simulink model "IMPexample2sim"  (R2018a)
settings: Solver=VariableStepAuto  StartTime=0.0  StopTime=10.0  RelTol=1e-3
values from neighbouring files (symbols this model uses):
  Ao = [Ap-Bp*Kp-Jp*Cp zeros(size(Ap,1),size(Av,2));-Jv*Cp Av]    [IMPexample2.m]
  Bo = [Jp Bp;Jv zeros(size(Jv,1),size(Bp,2))]    [IMPexample2.m]
  Bpo = [Jp Bp]    [IMPexample2.m]
  Jp = acker(Ap',Cp',-100)'    [IMPexample2.m]    (also in IMPexample3.m)
  Jv = acker(Av',Cv',[-10 -10 -10 -10])'    [IMPexample2.m]    (also in IMPexample3.m = acker(Av',Cv',[-10 -10 -10])')
  K = [Kp Cv]    [IMPexample2.m]
  Kp = acker(Ap,Bp,-10)    [IMPexample2.m]    (also in IMPexample3.m)
  Kpre = 1/evalfr(T,0)    [IMPexample2.m]    (also in IMPexample3.m)
  ref = 70*2*pi/60    (= 7.33038285838)    [IMPexample.m]    (also in IMPexample2.m; IMPexample3.m)
  Ts = 0.01    [IMPexample.m]    (also in IMPexample2.m)
undefined symbols (not defined in the file or in its folder): Ao_, Ap, Ap_, Apo_, Av, Avo_, Bo_, Bp, Bp_, Bpo_, Bvo_, Co_, Cp, Cp_, Cpo_, Cv, Cvo_, DiscIntNeverNeededParam, Do_, Dpo_, Dvo_, Jp_, Kp_
libraries: simulink x2
settings Model: Creator=Tobias Scala  LastModifiedBy=Tobias Scala

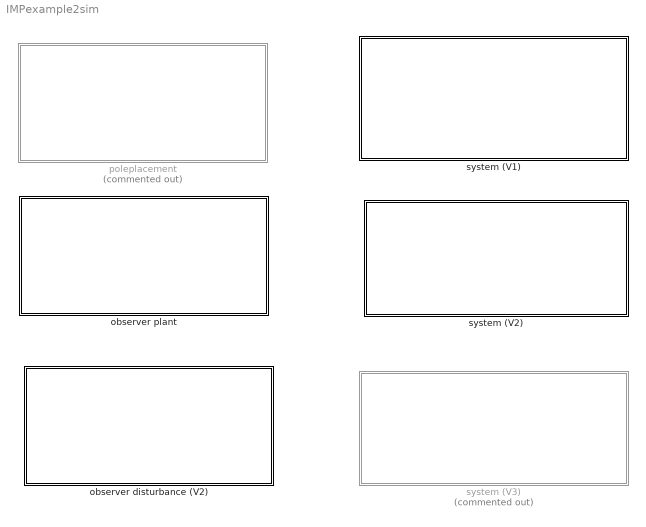
== system IMPexample2sim ==
  observer disturbance (V2) : Subsystem
  observer plant : Subsystem
  poleplacement : Subsystem  Commented=on
  system (V1) : Subsystem
  system (V2) : Subsystem
  system (V3) : Subsystem  Commented=on

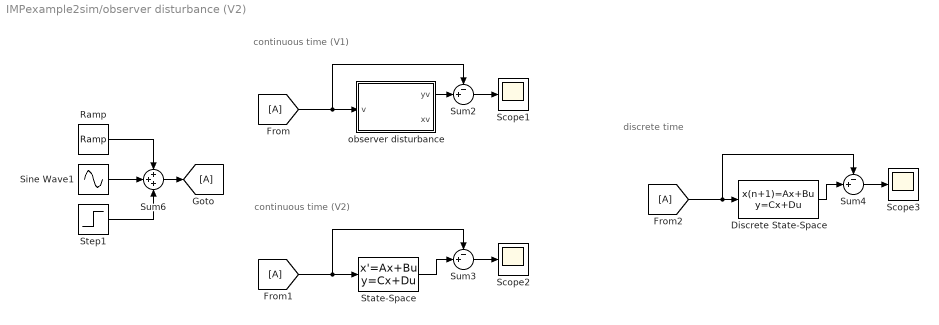
== system IMPexample2sim/observer disturbance (V2) ==
  note: discrete time
  note: continuous time (V2)
  note: continuous time (V1)
  Discrete State-Space : DiscreteStateSpace  A=Avo_  B=Bvo_  C=Cvo_  D=Dvo_  SampleTime=Ts
  Ramp : simulink/Sources/Ramp  slope=2  start=7  InitialOutput=0
  Scope1 : Scope
  Scope2 : Scope
  Scope3 : Scope
  Sine Wave1 : Sin  Amplitude=2  Frequency=2*ref  SampleTime=0
  State-Space : StateSpace  A=Av-Jv*Cv  B=Jv  C=Cv  D=zeros(size(Cv,1),size(Jv,2))  InitialCondition=0
  Step1 : Step  Time=4  After=2  SampleTime=0
  Sum2 : Sum  Inputs=-+|
  Sum3 : Sum  Inputs=-+|
  Sum4 : Sum  Inputs=-+|
  Sum6 : Sum  Inputs=+++
  observer disturbance : Subsystem
  wires:
  observer disturbance/1(yv) -> Sum2/2
  [A] -> observer disturbance/1(v), Sum2/1
  Sum2/1 -> Scope1/1
  Sum6/1 -> [A]
  [A] -> State-Space/1, Sum3/1
  State-Space/1 -> Sum3/2
  Sum3/1 -> Scope2/1
  Sum4/1 -> Scope3/1
  [A] -> Discrete State-Space/1, Sum4/1
  Discrete State-Space/1 -> Sum4/2
  Ramp/1 -> Sum6/1
  Step1/1 -> Sum6/3
  Sine Wave1/1 -> Sum6/2

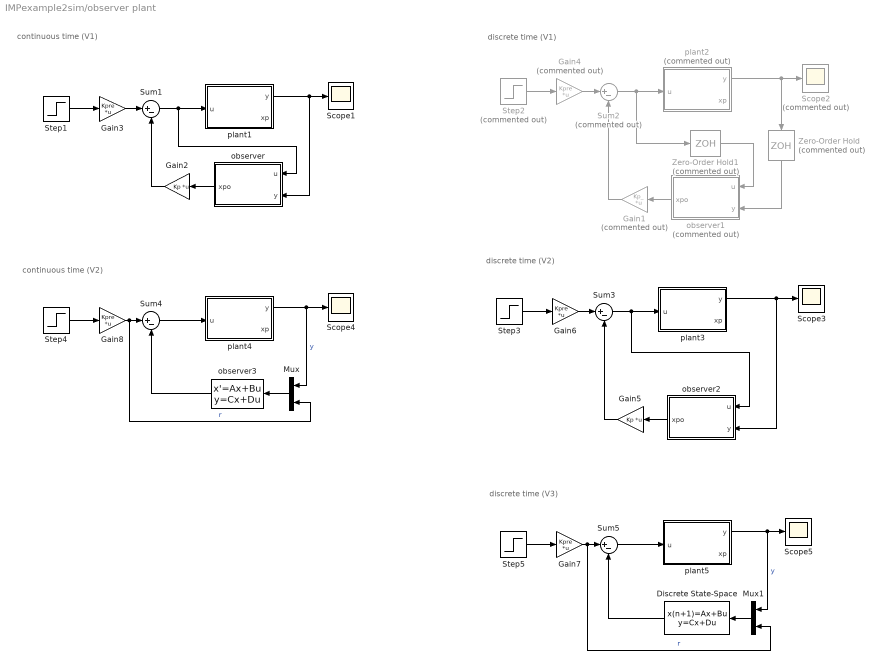
== system IMPexample2sim/observer plant ==
  note: discrete time (V3)
  note: continuous time (V2)
  note: discrete time (V2)
  note: discrete time (V1)
  note: continuous time (V1)
  Discrete State-Space : DiscreteStateSpace  A=Apo_  B=Bpo_  C=Cpo_  D=Dpo_  SampleTime=Ts
  Gain1 : Gain  Commented=on  Gain=Kp_  Multiplication=Matrix(K*u)
  Gain2 : Gain  Gain=Kp  Multiplication=Matrix(K*u)
  Gain{3,6..8} (4 alike) : Gain  Gain=Kpre  Multiplication=Matrix(K*u)
  Gain4 : Gain  Commented=on  Gain=Kpre  Multiplication=Matrix(K*u)
  Gain5 : Gain  Gain=Kp  Multiplication=Matrix(K*u)
  Mux : Mux  Inputs=2
  Mux1 : Mux  Inputs=2
  Scope{1,3..5} (4 alike) : Scope
  Scope2 : Scope  Commented=on
  Step{1,3..5} (4 alike) : Step  After=ref  SampleTime=0
  Step2 : Step  Commented=on  After=ref  SampleTime=0
  Sum{1,3..5} (4 alike) : Sum  Inputs=|+-
  Sum2 : Sum  Commented=on  Inputs=|+-
  Zero-Order Hold : ZeroOrderHold  Commented=on  SampleTime=Ts
  Zero-Order Hold1 : ZeroOrderHold  Commented=on  SampleTime=Ts
  observer : Subsystem
  observer1 : Subsystem  Commented=on
  observer2 : Subsystem
  observer3 : StateSpace  A=Ap-Bp*Kp-Jp*Cp  B=Bpo  C=Kp  D=zeros(size(Kp,1),size(Bpo,2))  InitialCondition=0
  plant1 : Subsystem
  plant2 : Subsystem  Commented=on
  plant3 : Subsystem
  plant4 : Subsystem
  plant5 : Subsystem
  wires:
  plant1/1(y) -> observer/2(y), Scope1/1
  Sum1/1 -> plant1/1(u), observer/1(u)
  Gain3/1 -> Sum1/1
  Step1/1 -> Gain3/1
  Gain2/1 -> Sum1/2
  observer/1(xpo) -> Gain2/1
  observer1/1(xpo) -> Gain1/1
  plant2/1(y) -> Zero-Order Hold/1, Scope2/1
  Step2/1 -> Gain4/1
  Gain4/1 -> Sum2/1
  Sum2/1 -> plant2/1(u), Zero-Order Hold1/1
  Gain1/1 -> Sum2/2
  Zero-Order Hold/1 -> observer1/2(y)
  Zero-Order Hold1/1 -> observer1/1(u)
  plant3/1(y) -> observer2/2(y), Scope3/1
  observer2/1(xpo) -> Gain5/1
  Gain5/1 -> Sum3/2
  Sum3/1 -> observer2/1(u), plant3/1(u)
  Step3/1 -> Gain6/1
  Gain6/1 -> Sum3/1
  observer3/1 -> Sum4/2
  Sum4/1 -> plant4/1(u)
  Gain8/1 -> Mux/2, Sum4/1  "r"
  Step4/1 -> Gain8/1
  plant4/1(y) -> Mux/1, Scope4/1  "y"
  plant5/1(y) -> Scope5/1, Mux1/1  "y"
  Step5/1 -> Gain7/1
  Gain7/1 -> Mux1/2, Sum5/1  "r"
  Sum5/1 -> plant5/1(u)
  Discrete State-Space/1 -> Sum5/2
  Mux/1 -> observer3/1
  Mux1/1 -> Discrete State-Space/1

== system IMPexample2sim/poleplacement ==
  Gain : Gain  Gain=Kp  Multiplication=Matrix(K*u)
  Gain1 : Gain  Gain=Kpre  Multiplication=Matrix(K*u)
  Scope : Scope
  Step : Step  After=ref  SampleTime=0
  Sum : Sum  Inputs=|+-
  plant : Subsystem
  wires:
  Step/1 -> Gain1/1
  plant/2(xp) -> Gain/1
  Gain1/1 -> Sum/1
  Sum/1 -> plant/1(u)
  Gain/1 -> Sum/2
  plant/1(yp) -> Scope/1

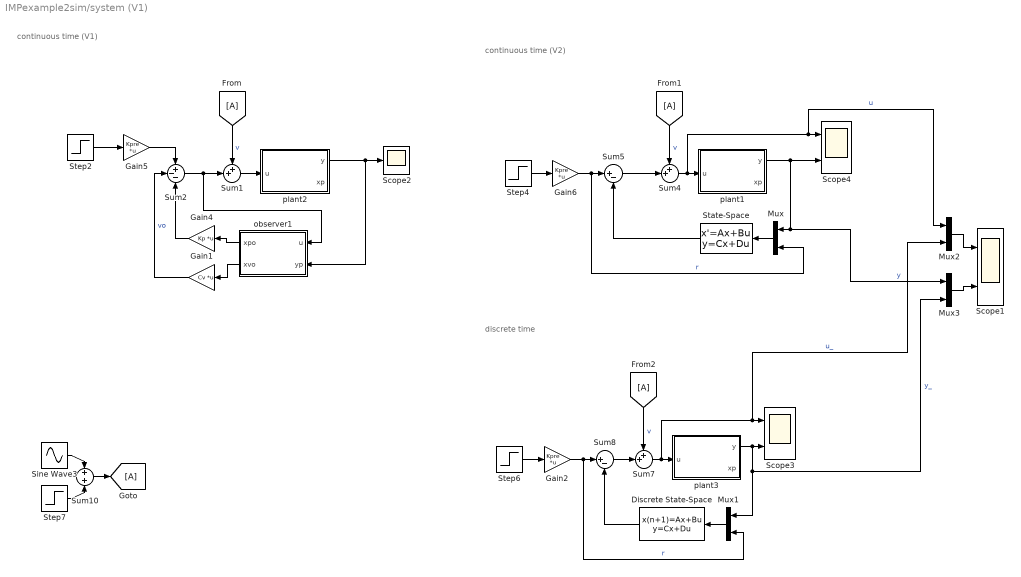
== system IMPexample2sim/system (V1) ==
  note: discrete time
  note: continuous time (V2)
  note: continuous time (V1)
  Discrete State-Space : DiscreteStateSpace  A=Ao_  B=Bo_  C=Co_  D=Do_  SampleTime=Ts
  Gain1 : Gain  Gain=Cv  Multiplication=Matrix(K*u)
  Gain2 : Gain  Gain=Kpre  Multiplication=Matrix(K*u)
  Gain4 : Gain  Gain=Kp  Multiplication=Matrix(K*u)
  Gain5 : Gain  Gain=Kpre  Multiplication=Matrix(K*u)
  Gain6 : Gain  Gain=Kpre  Multiplication=Matrix(K*u)
  Mux{,1..3} (4 alike) : Mux  Inputs=2
  Scope1 : Scope  NumInputPorts=2
  Scope2 : Scope
  Scope3 : Scope  NumInputPorts=2
  Scope4 : Scope  NumInputPorts=2
  Sine Wave3 : Sin  Amplitude=2  Frequency=2*ref  SampleTime=0
  State-Space : StateSpace  A=Ao  B=Bo  C=K  D=zeros(size(K,1),size(Bo,2))  InitialCondition=0
  Step2 : Step  After=ref  SampleTime=0
  Step4 : Step  After=ref  SampleTime=0
  Step6 : Step  After=ref  SampleTime=0
  Step7 : Step  Time=4  After=2  SampleTime=0
  Sum1 : Sum  Inputs=++|
  Sum10 : Sum  Inputs=+|+
  Sum2 : Sum  Inputs=+--
  Sum4 : Sum  Inputs=++|
  Sum5 : Sum  Inputs=|+-
  Sum7 : Sum  Inputs=++|
  Sum8 : Sum  Inputs=|+-
  observer1 : Subsystem
  plant1 : Subsystem
  plant2 : Subsystem
  plant3 : Subsystem
  wires:
  plant2/1(y) -> observer1/2(yp), Scope2/1
  Sum1/1 -> plant2/1(u)
  Gain1/1 -> Sum2/2  "vo"
  [A] -> Sum1/1  "v"
  Sum2/1 -> Sum1/2, observer1/1(u)
  observer1/2(xvo) -> Gain1/1
  Step2/1 -> Gain5/1
  Gain4/1 -> Sum2/3
  observer1/1(xpo) -> Gain4/1
  Gain5/1 -> Sum2/1
  [A] -> Sum4/1  "v"
  Sum5/1 -> Sum4/2
  State-Space/1 -> Sum5/2
  plant1/1(y) -> Mux3/1, Mux/1, Scope4/2  "y"
  Step4/1 -> Gain6/1
  Sum4/1 -> Mux2/1, Scope4/1, plant1/1(u)  "u"
  Gain6/1 -> Mux/2, Sum5/1  "r"
  Mux/1 -> State-Space/1
  Discrete State-Space/1 -> Sum8/2
  Step6/1 -> Gain2/1
  Gain2/1 -> Mux1/2, Sum8/1  "r"
  Sum7/1 -> Mux2/2, Scope3/1, plant3/1(u)  "u_"
  [A] -> Sum7/1  "v"
  plant3/1(y) -> Mux3/2, Mux1/1, Scope3/2  "y_"
  Mux1/1 -> Discrete State-Space/1
  Sum8/1 -> Sum7/2
  Mux2/1 -> Scope1/1
  Mux3/1 -> Scope1/2
  Step7/1 -> Sum10/2
  Sum10/1 -> [A]
  Sine Wave3/1 -> Sum10/1

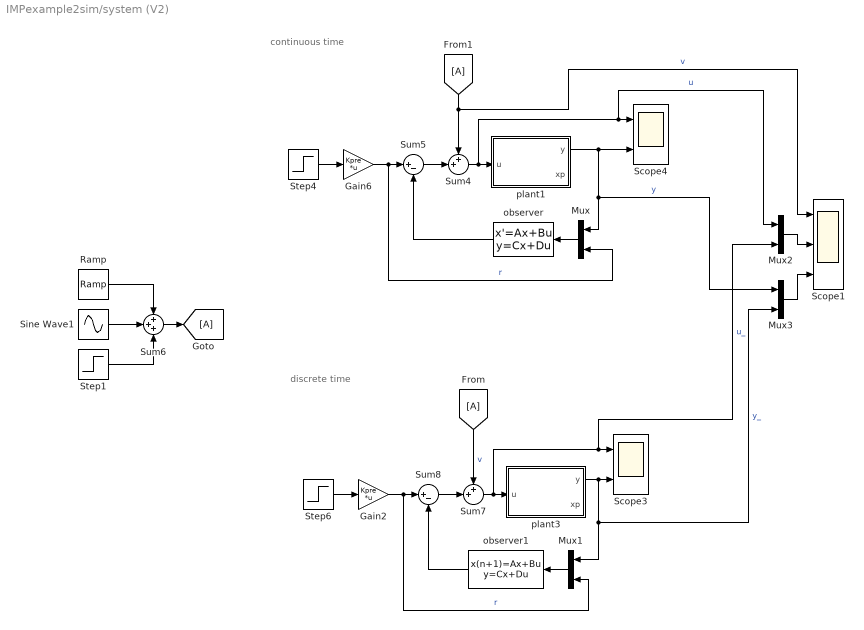
== system IMPexample2sim/system (V2) ==
  note: discrete time
  note: continuous time
  Gain2 : Gain  Gain=Kpre  Multiplication=Matrix(K*u)
  Gain6 : Gain  Gain=Kpre  Multiplication=Matrix(K*u)
  Mux{,1..3} (4 alike) : Mux  Inputs=2
  Ramp : simulink/Sources/Ramp  slope=2  start=7  InitialOutput=0
  Scope1 : Scope  NumInputPorts=3
  Scope3 : Scope  NumInputPorts=2
  Scope4 : Scope  NumInputPorts=2
  Sine Wave1 : Sin  Amplitude=2  Frequency=2*ref  SampleTime=0
  Step1 : Step  Time=4  After=2  SampleTime=0
  Step4 : Step  After=ref  SampleTime=0
  Step6 : Step  After=ref  SampleTime=0
  Sum4 : Sum  Inputs=++|
  Sum5 : Sum  Inputs=|+-
  Sum6 : Sum  Inputs=+++
  Sum7 : Sum  Inputs=++|
  Sum8 : Sum  Inputs=|+-
  observer : StateSpace  A=Ao  B=Bo  C=K  D=zeros(size(K,1),size(Bo,2))  InitialCondition=0
  observer1 : DiscreteStateSpace  A=Ao_  B=Bo_  C=Co_  D=Do_  SampleTime=Ts
  plant1 : Subsystem
  plant3 : Subsystem
  wires:
  Sum7/1 -> Mux2/2, Scope3/1, plant3/1(u)  "u_"
  [A] -> Sum4/1, Scope1/1  "v"
  Sum5/1 -> Sum4/2
  Step6/1 -> Gain2/1
  Mux/1 -> observer/1
  plant1/1(y) -> Mux/1, Mux3/1, Scope4/2  "y"
  plant3/1(y) -> Mux3/2, Mux1/1, Scope3/2  "y_"
  Gain6/1 -> Mux/2, Sum5/1  "r"
  [A] -> Sum7/1  "v"
  observer1/1 -> Sum8/2
  observer/1 -> Sum5/2
  Sum8/1 -> Sum7/2
  Step4/1 -> Gain6/1
  Sum4/1 -> Mux2/1, Scope4/1, plant1/1(u)  "u"
  Mux3/1 -> Scope1/3
  Mux2/1 -> Scope1/2
  Mux1/1 -> observer1/1
  Gain2/1 -> Mux1/2, Sum8/1  "r"
  Step1/1 -> Sum6/3
  Sine Wave1/1 -> Sum6/2
  Ramp/1 -> Sum6/1
  Sum6/1 -> [A]

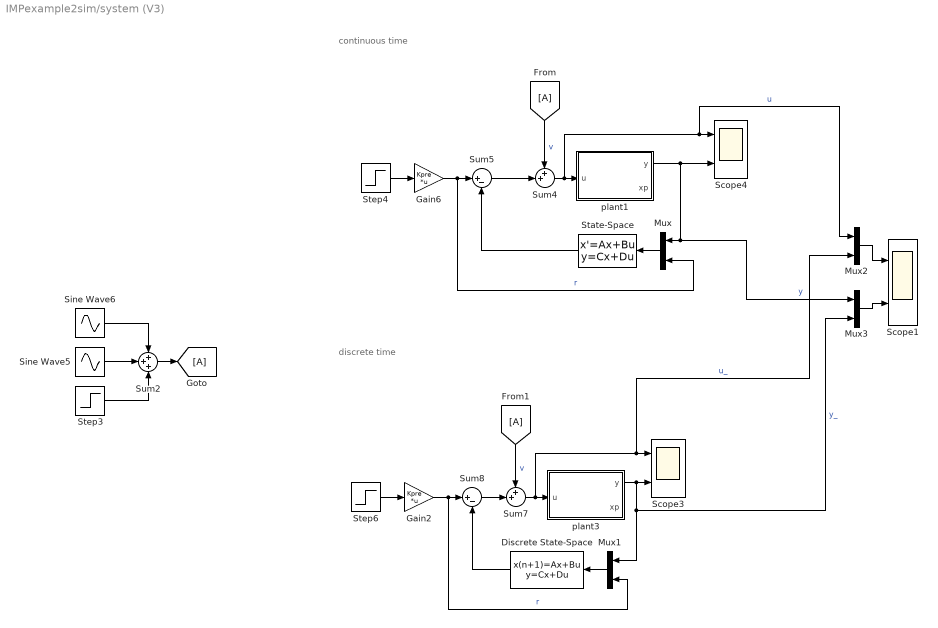
== system IMPexample2sim/system (V3) ==
  note: discrete time
  note: continuous time
  Discrete State-Space : DiscreteStateSpace  A=Ao_  B=Bo_  C=Co_  D=Do_  SampleTime=Ts
  Gain2 : Gain  Gain=Kpre  Multiplication=Matrix(K*u)
  Gain6 : Gain  Gain=Kpre  Multiplication=Matrix(K*u)
  Mux{,1..3} (4 alike) : Mux  Inputs=2
  Scope1 : Scope  NumInputPorts=2
  Scope3 : Scope  NumInputPorts=2
  Scope4 : Scope  NumInputPorts=2
  Sine Wave5 : Sin  Amplitude=2  Frequency=2*ref  SampleTime=0
  Sine Wave6 : Sin  Frequency=4*ref  SampleTime=0
  State-Space : StateSpace  A=Ao  B=Bo  C=K  D=zeros(size(K,1),size(Bo,2))  InitialCondition=0
  Step3 : Step  Time=4  After=2  SampleTime=0
  Step4 : Step  After=ref  SampleTime=0
  Step6 : Step  After=ref  SampleTime=0
  Sum2 : Sum  Inputs=+++
  Sum4 : Sum  Inputs=++|
  Sum5 : Sum  Inputs=|+-
  Sum7 : Sum  Inputs=++|
  Sum8 : Sum  Inputs=|+-
  plant1 : Subsystem
  plant3 : Subsystem
  wires:
  plant3/1(y) -> Mux3/2, Mux1/1, Scope3/2  "y_"
  State-Space/1 -> Sum5/2
  Gain6/1 -> Mux/2, Sum5/1  "r"
  Sum4/1 -> Mux2/1, Scope4/1, plant1/1(u)  "u"
  Sum7/1 -> Mux2/2, Scope3/1, plant3/1(u)  "u_"
  Mux/1 -> State-Space/1
  Step6/1 -> Gain2/1
  plant1/1(y) -> Mux3/1, Mux/1, Scope4/2  "y"
  Step4/1 -> Gain6/1
  [A] -> Sum4/1  "v"
  Gain2/1 -> Mux1/2, Sum8/1  "r"
  Sum5/1 -> Sum4/2
  Discrete State-Space/1 -> Sum8/2
  Mux1/1 -> Discrete State-Space/1
  [A] -> Sum7/1  "v"
  Sum8/1 -> Sum7/2
  Mux3/1 -> Scope1/2
  Mux2/1 -> Scope1/1
  Sine Wave6/1 -> Sum2/1
  Step3/1 -> Sum2/3
  Sum2/1 -> [A]
  Sine Wave5/1 -> Sum2/2

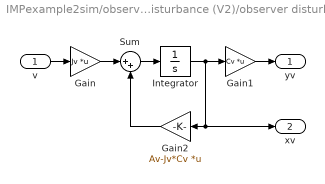
== system IMPexample2sim/observer disturbance (V2)/observer disturbance ==
  v : Inport
  Gain : Gain  Gain=Jv  Multiplication=Matrix(K*u)
  Gain1 : Gain  Gain=Cv  Multiplication=Matrix(K*u)
  Gain2 : Gain  Gain=Av-Jv*Cv  Multiplication=Matrix(K*u)
  Integrator : Integrator
  Sum : Sum  Inputs=|++
  yv : Outport
  xv : Outport  Port=2
  wires:
  Gain1/1 -> yv/1
  Gain/1 -> Sum/1
  Gain2/1 -> Sum/2
  v/1 -> Gain/1
  Sum/1 -> Integrator/1
  Integrator/1 -> xv/1, Gain2/1, Gain1/1

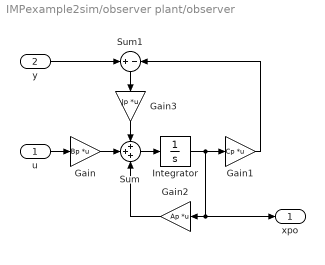
== system IMPexample2sim/observer plant/observer ==
  u : Inport
  y : Inport  Port=2
  Gain : Gain  Gain=Bp  Multiplication=Matrix(K*u)
  Gain1 : Gain  Gain=Cp  Multiplication=Matrix(K*u)
  Gain2 : Gain  Gain=Ap  Multiplication=Matrix(K*u)
  Gain3 : Gain  Gain=Jp  Multiplication=Matrix(K*u)
  Integrator : Integrator
  Sum : Sum  Inputs=+++
  Sum1 : Sum  Inputs=+|-
  xpo : Outport
  wires:
  Gain1/1 -> Sum1/2
  u/1 -> Gain/1
  Sum/1 -> Integrator/1
  Integrator/1 -> xpo/1, Gain2/1, Gain1/1
  Gain/1 -> Sum/2
  Gain2/1 -> Sum/3
  y/1 -> Sum1/1
  Sum1/1 -> Gain3/1
  Gain3/1 -> Sum/1

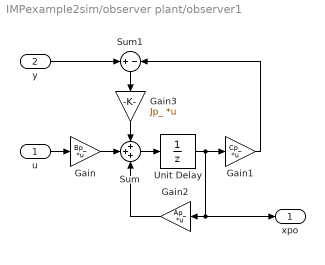
== system IMPexample2sim/observer plant/observer1 ==
  u : Inport
  y : Inport  Port=2
  Gain : Gain  Gain=Bp_  Multiplication=Matrix(K*u)
  Gain1 : Gain  Gain=Cp_  Multiplication=Matrix(K*u)
  Gain2 : Gain  Gain=Ap_  Multiplication=Matrix(K*u)
  Gain3 : Gain  Gain=Jp_  Multiplication=Matrix(K*u)
  Sum : Sum  Inputs=+++
  Sum1 : Sum  Inputs=+|-
  Unit Delay : UnitDelay  SampleTime=Ts
  xpo : Outport
  wires:
  Gain1/1 -> Sum1/2
  u/1 -> Gain/1
  Sum/1 -> Unit Delay/1
  Unit Delay/1 -> xpo/1, Gain2/1, Gain1/1
  Gain/1 -> Sum/2
  Gain2/1 -> Sum/3
  y/1 -> Sum1/1
  Sum1/1 -> Gain3/1
  Gain3/1 -> Sum/1

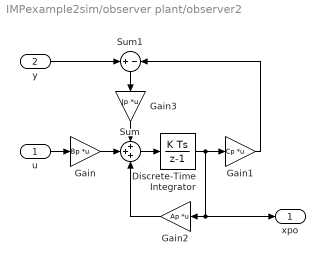
== system IMPexample2sim/observer plant/observer2 ==
  u : Inport
  y : Inport  Port=2
  Discrete-Time Integrator : DiscreteIntegrator  SampleTime=0.01  ICPrevOutput=DiscIntNeverNeededParam  ICPrevScaledInput=DiscIntNeverNeededParam
  Gain : Gain  Gain=Bp  Multiplication=Matrix(K*u)
  Gain1 : Gain  Gain=Cp  Multiplication=Matrix(K*u)
  Gain2 : Gain  Gain=Ap  Multiplication=Matrix(K*u)
  Gain3 : Gain  Gain=Jp  Multiplication=Matrix(K*u)
  Sum : Sum  Inputs=+++
  Sum1 : Sum  Inputs=+|-
  xpo : Outport
  wires:
  Gain1/1 -> Sum1/2
  u/1 -> Gain/1
  Sum/1 -> Discrete-Time Integrator/1
  Discrete-Time Integrator/1 -> xpo/1, Gain2/1, Gain1/1
  Gain/1 -> Sum/2
  Gain2/1 -> Sum/3
  y/1 -> Sum1/1
  Sum1/1 -> Gain3/1
  Gain3/1 -> Sum/1

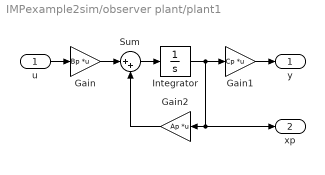
== system IMPexample2sim/observer plant/plant1 ==
  u : Inport
  Gain : Gain  Gain=Bp  Multiplication=Matrix(K*u)
  Gain1 : Gain  Gain=Cp  Multiplication=Matrix(K*u)
  Gain2 : Gain  Gain=Ap  Multiplication=Matrix(K*u)
  Integrator : Integrator
  Sum : Sum  Inputs=|++
  y : Outport
  xp : Outport  Port=2
  wires:
  Gain1/1 -> y/1
  Gain/1 -> Sum/1
  Gain2/1 -> Sum/2
  u/1 -> Gain/1
  Sum/1 -> Integrator/1
  Integrator/1 -> xp/1, Gain2/1, Gain1/1

== system IMPexample2sim/observer plant/plant2 ==
  u : Inport
  Gain : Gain  Gain=Bp  Multiplication=Matrix(K*u)
  Gain1 : Gain  Gain=Cp  Multiplication=Matrix(K*u)
  Gain2 : Gain  Gain=Ap  Multiplication=Matrix(K*u)
  Integrator : Integrator
  Sum : Sum  Inputs=|++
  y : Outport
  xp : Outport  Port=2
  wires:
  Gain1/1 -> y/1
  Gain/1 -> Sum/1
  Gain2/1 -> Sum/2
  u/1 -> Gain/1
  Sum/1 -> Integrator/1
  Integrator/1 -> xp/1, Gain2/1, Gain1/1

== system IMPexample2sim/observer plant/plant3 ==
  u : Inport
  Gain : Gain  Gain=Bp  Multiplication=Matrix(K*u)
  Gain1 : Gain  Gain=Cp  Multiplication=Matrix(K*u)
  Gain2 : Gain  Gain=Ap  Multiplication=Matrix(K*u)
  Integrator : Integrator
  Sum : Sum  Inputs=|++
  y : Outport
  xp : Outport  Port=2
  wires:
  Gain1/1 -> y/1
  Gain/1 -> Sum/1
  Gain2/1 -> Sum/2
  u/1 -> Gain/1
  Sum/1 -> Integrator/1
  Integrator/1 -> xp/1, Gain2/1, Gain1/1

== system IMPexample2sim/observer plant/plant4 ==
  u : Inport
  Gain : Gain  Gain=Bp  Multiplication=Matrix(K*u)
  Gain1 : Gain  Gain=Cp  Multiplication=Matrix(K*u)
  Gain2 : Gain  Gain=Ap  Multiplication=Matrix(K*u)
  Integrator : Integrator
  Sum : Sum  Inputs=|++
  y : Outport
  xp : Outport  Port=2
  wires:
  Gain1/1 -> y/1
  Gain/1 -> Sum/1
  Gain2/1 -> Sum/2
  u/1 -> Gain/1
  Sum/1 -> Integrator/1
  Integrator/1 -> xp/1, Gain2/1, Gain1/1

== system IMPexample2sim/observer plant/plant5 ==
  u : Inport
  Gain : Gain  Gain=Bp  Multiplication=Matrix(K*u)
  Gain1 : Gain  Gain=Cp  Multiplication=Matrix(K*u)
  Gain2 : Gain  Gain=Ap  Multiplication=Matrix(K*u)
  Integrator : Integrator
  Sum : Sum  Inputs=|++
  y : Outport
  xp : Outport  Port=2
  wires:
  Gain1/1 -> y/1
  Gain/1 -> Sum/1
  Gain2/1 -> Sum/2
  u/1 -> Gain/1
  Sum/1 -> Integrator/1
  Integrator/1 -> xp/1, Gain2/1, Gain1/1

== system IMPexample2sim/poleplacement/plant ==
  u : Inport
  Gain : Gain  Gain=Bp  Multiplication=Matrix(K*u)
  Gain1 : Gain  Gain=Cp  Multiplication=Matrix(K*u)
  Gain2 : Gain  Gain=Ap  Multiplication=Matrix(K*u)
  Integrator : Integrator
  Sum : Sum  Inputs=|++
  yp : Outport
  xp : Outport  Port=2
  wires:
  Gain1/1 -> yp/1
  Gain/1 -> Sum/1
  Gain2/1 -> Sum/2
  u/1 -> Gain/1
  Sum/1 -> Integrator/1
  Integrator/1 -> xp/1, Gain2/1, Gain1/1

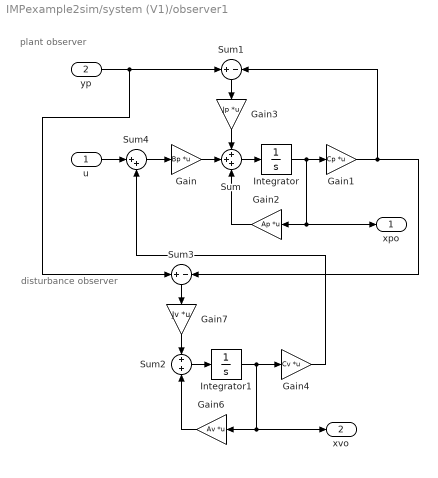
== system IMPexample2sim/system (V1)/observer1 ==
  note: disturbance observer
  note: plant observer
  u : Inport
  yp : Inport  Port=2
  Gain : Gain  Gain=Bp  Multiplication=Matrix(K*u)
  Gain1 : Gain  Gain=Cp  Multiplication=Matrix(K*u)
  Gain2 : Gain  Gain=Ap  Multiplication=Matrix(K*u)
  Gain3 : Gain  Gain=Jp  Multiplication=Matrix(K*u)
  Gain4 : Gain  Gain=Cv  Multiplication=Matrix(K*u)
  Gain6 : Gain  Gain=Av  Multiplication=Matrix(K*u)
  Gain7 : Gain  Gain=Jv  Multiplication=Matrix(K*u)
  Integrator : Integrator
  Integrator1 : Integrator
  Sum : Sum  Inputs=+++
  Sum1 : Sum  Inputs=+|-
  Sum2 : Sum  Inputs=+|+
  Sum3 : Sum  Inputs=+|-
  Sum4 : Sum  Inputs=|++
  xpo : Outport
  xvo : Outport  Port=2
  wires:
  Gain1/1 -> Sum3/2, Sum1/2
  u/1 -> Sum4/1
  Sum/1 -> Integrator/1
  Integrator/1 -> xpo/1, Gain2/1, Gain1/1
  Gain/1 -> Sum/2
  Gain2/1 -> Sum/3
  Sum1/1 -> Gain3/1
  Gain3/1 -> Sum/1
  yp/1 -> Sum3/1, Sum1/1
  Sum3/1 -> Gain7/1
  Gain6/1 -> Sum2/2
  Sum2/1 -> Integrator1/1
  Gain7/1 -> Sum2/1
  Integrator1/1 -> Gain4/1, xvo/1, Gain6/1
  Sum4/1 -> Gain/1
  Gain4/1 -> Sum4/2

== system IMPexample2sim/system (V1)/plant1 ==
  u : Inport
  Gain : Gain  Gain=Bp  Multiplication=Matrix(K*u)
  Gain1 : Gain  Gain=Cp  Multiplication=Matrix(K*u)
  Gain2 : Gain  Gain=Ap  Multiplication=Matrix(K*u)
  Integrator : Integrator
  Sum : Sum  Inputs=|++
  y : Outport
  xp : Outport  Port=2
  wires:
  Gain1/1 -> y/1
  Gain/1 -> Sum/1
  Gain2/1 -> Sum/2
  u/1 -> Gain/1
  Sum/1 -> Integrator/1
  Integrator/1 -> xp/1, Gain2/1, Gain1/1

== system IMPexample2sim/system (V1)/plant2 ==
  u : Inport
  Gain : Gain  Gain=Bp  Multiplication=Matrix(K*u)
  Gain1 : Gain  Gain=Cp  Multiplication=Matrix(K*u)
  Gain2 : Gain  Gain=Ap  Multiplication=Matrix(K*u)
  Integrator : Integrator
  Sum : Sum  Inputs=|++
  y : Outport
  xp : Outport  Port=2
  wires:
  Gain1/1 -> y/1
  Gain/1 -> Sum/1
  Gain2/1 -> Sum/2
  u/1 -> Gain/1
  Sum/1 -> Integrator/1
  Integrator/1 -> xp/1, Gain2/1, Gain1/1

== system IMPexample2sim/system (V1)/plant3 ==
  u : Inport
  Gain : Gain  Gain=Bp  Multiplication=Matrix(K*u)
  Gain1 : Gain  Gain=Cp  Multiplication=Matrix(K*u)
  Gain2 : Gain  Gain=Ap  Multiplication=Matrix(K*u)
  Integrator : Integrator
  Sum : Sum  Inputs=|++
  y : Outport
  xp : Outport  Port=2
  wires:
  Gain1/1 -> y/1
  Gain/1 -> Sum/1
  Gain2/1 -> Sum/2
  u/1 -> Gain/1
  Sum/1 -> Integrator/1
  Integrator/1 -> xp/1, Gain2/1, Gain1/1

== system IMPexample2sim/system (V2)/plant1 ==
  u : Inport
  Gain : Gain  Gain=Bp  Multiplication=Matrix(K*u)
  Gain1 : Gain  Gain=Cp  Multiplication=Matrix(K*u)
  Gain2 : Gain  Gain=Ap  Multiplication=Matrix(K*u)
  Integrator : Integrator
  Sum : Sum  Inputs=|++
  y : Outport
  xp : Outport  Port=2
  wires:
  Gain1/1 -> y/1
  Gain/1 -> Sum/1
  Gain2/1 -> Sum/2
  u/1 -> Gain/1
  Sum/1 -> Integrator/1
  Integrator/1 -> xp/1, Gain2/1, Gain1/1

== system IMPexample2sim/system (V2)/plant3 ==
  u : Inport
  Gain : Gain  Gain=Bp  Multiplication=Matrix(K*u)
  Gain1 : Gain  Gain=Cp  Multiplication=Matrix(K*u)
  Gain2 : Gain  Gain=Ap  Multiplication=Matrix(K*u)
  Integrator : Integrator
  Sum : Sum  Inputs=|++
  y : Outport
  xp : Outport  Port=2
  wires:
  Gain1/1 -> y/1
  Gain/1 -> Sum/1
  Gain2/1 -> Sum/2
  u/1 -> Gain/1
  Sum/1 -> Integrator/1
  Integrator/1 -> xp/1, Gain2/1, Gain1/1

== system IMPexample2sim/system (V3)/plant1 ==
  u : Inport
  Gain : Gain  Gain=Bp  Multiplication=Matrix(K*u)
  Gain1 : Gain  Gain=Cp  Multiplication=Matrix(K*u)
  Gain2 : Gain  Gain=Ap  Multiplication=Matrix(K*u)
  Integrator : Integrator
  Sum : Sum  Inputs=|++
  y : Outport
  xp : Outport  Port=2
  wires:
  Gain1/1 -> y/1
  Gain/1 -> Sum/1
  Gain2/1 -> Sum/2
  u/1 -> Gain/1
  Sum/1 -> Integrator/1
  Integrator/1 -> xp/1, Gain2/1, Gain1/1

== system IMPexample2sim/system (V3)/plant3 ==
  u : Inport
  Gain : Gain  Gain=Bp  Multiplication=Matrix(K*u)
  Gain1 : Gain  Gain=Cp  Multiplication=Matrix(K*u)
  Gain2 : Gain  Gain=Ap  Multiplication=Matrix(K*u)
  Integrator : Integrator
  Sum : Sum  Inputs=|++
  y : Outport
  xp : Outport  Port=2
  wires:
  Gain1/1 -> y/1
  Gain/1 -> Sum/1
  Gain2/1 -> Sum/2
  u/1 -> Gain/1
  Sum/1 -> Integrator/1
  Integrator/1 -> xp/1, Gain2/1, Gain1/1
